simulink model "Intretesatoare"  (R2016a)
settings: Solver=VariableStepAuto  StartTime=0.0  StopTime=100  RelTol=1e-3
values from neighbouring files (symbols this model uses):
  a = floor(sqrt(data.BlockLength))    [BERPerformance3.m]    (also in Interleaver.m = floor(sqrt(BlockLength)))
  b = b+1    [BERPerformance3.m]    (also in Interleaver.m; Perioada_Repetitie.m = reshape(Secventa_Generata(1:(m*floor(length(Secventa_Generat)
  BlockLength = [128 4096]    [BERPerformance.m]    (also in DistantaMinima.m = length(si); Interleaver.m = str2double(answer{1}); Top.m = str2double(answer{1}))
  Date = (1:data.BlockLength)    [BERPerformance3.m]    (also in Interleaver.m = 1:BlockLength)
  Index = unique(Secventa_Generata,'stable')'+1    [Interleaver.m]
libraries: commblkintrlv2 x3, dspsigops x1
settings Model: Creator=Orza  LastModifiedBy=Orza
settings DataIOCC: SaveTime=off

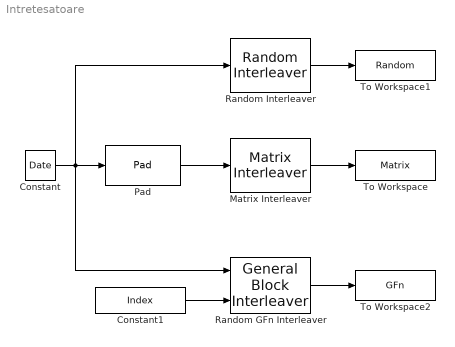
== system Intretesatoare ==
  Constant : Constant  Value=Date
  Constant1 : Constant  Value=Index
  Matrix Interleaver : commblkintrlv2/Matrix Interleaver  Nrows=a  Ncols=b
  Pad : dspsigops/Pad  padAlong=Columns  dimsToPad=1  valSrc=Specify via dialog  padVal=0  spec=Output size  padNumOutRowsSpecMethod=User-specified  numOutRows=a*b  padNumOutColsSpecMethod=User-specified  numOutCols=1  isVarDimsMode=off  padBeginning=0  padEnd=0  outSizeMode=User-specified  outSize=1  padSigAt=End  trunc_flag=None  roundingMode=Floor  overflowMode=off  truncOrWrapMode=Truncate  wrap_flag=None
  Random Interleaver : commblkintrlv2/Random Interleaver  N=BlockLength  seed=12345
  Random GFn Interleaver : commblkintrlv2/General Block Interleaver  permutationVectorSource=Input port  elements=[5:-1:1].'
  To Workspace : ToWorkspace  VariableName=Matrix  SampleTime=-1
      settings: MaxDataPoints=1  Save2DSignal=2-D array (concatenate along first dimension)
  To Workspace1 : ToWorkspace  VariableName=Random  SampleTime=-1
      settings: MaxDataPoints=1  Save2DSignal=2-D array (concatenate along first dimension)
  To Workspace2 : ToWorkspace  VariableName=GFn  SampleTime=-1
      settings: MaxDataPoints=1  Save2DSignal=2-D array (concatenate along first dimension)
  wires:
  Constant/1 -> Random GFn Interleaver/1, Random Interleaver/1, Pad/1
  Pad/1 -> Matrix Interleaver/1
  Matrix Interleaver/1 -> To Workspace/1
  Random Interleaver/1 -> To Workspace1/1
  Constant1/1 -> Random GFn Interleaver/2
  Random GFn Interleaver/1 -> To Workspace2/1
